simulink model "Arc_Trajectory_Sim"  (R2026a)
settings: Solver=VariableStepAuto  StopTime=5.0
settings Model: Creator=shueb  LastModifiedBy=shueb

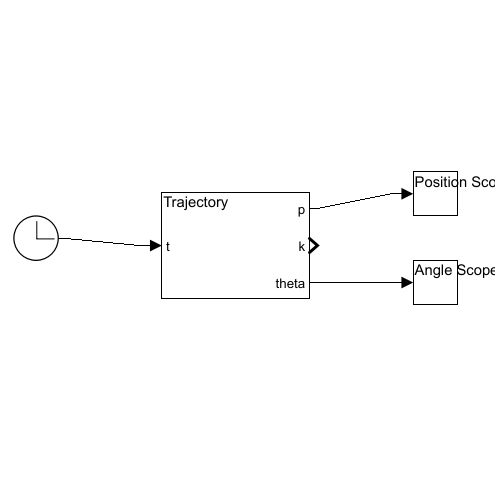
[thumbnail: Simulink's stored preview of the top-level diagram]
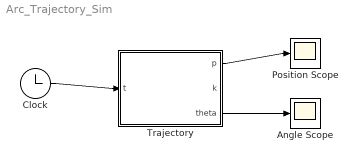
== system Arc_Trajectory_Sim ==
  Angle Scope : Scope
  Clock : Clock
  Position Scope : Scope
  Trajectory : MATLAB Function  TreatAsAtomicUnit=on
  wires:
  Clock/1 -> Trajectory/1(t)
  Trajectory/1(p) -> Position Scope/1
  Trajectory/3(theta) -> Angle Scope/1

== matlab function Arc_Trajectory_Sim/Trajectory ==
  data: t input; p output; k output; theta output
function [p, k, theta] = fcn(t)
    % Trajectory parameters
    tf = 5;
    R = 1;

    % Cubic timing law
    if t <= 0
        s = 0;
    elseif t >= tf
        s = 1;
    else
        s = 3*(t/tf)^2 - 2*(t/tf)^3;
    end

    % Angle along the arc
    phi = (pi/2) * s;

    % Position [x; y; z]
    p = [0; R*sin(phi); R*cos(phi)];

    % Orientation (Vector-Angle)
    k = [-1; 0; 0];
    theta = phi;
end
